simulink model "Dyn_Nonlinear_four"  (R2021a)
(part 4 of 7)

C(5,3) = 0.056*thetad2*cos(theta5)^2 - 0.028*thetad3 - 0.028*thetad4 - 0.028*thetad2 + 0.056*thetad3*cos(theta5)^2 + 0.056*thetad4*cos(theta5)^2 - 0.0098*thetad5*cos(theta5) + 0.049*thetad5*sin(theta5) + 0.14*thetad2*cos(theta4)*cos(theta5) + 0.14*thetad3*cos(theta4)*cos(theta5) + 0.07*thetad4*cos(theta4)*cos(theta5) + 0.028*thetad2*cos(theta4)*sin(theta5) - 0.1344*thetad2*cos(theta5)*sin(theta5) + 0.028*thetad3*cos(theta4)*sin(theta5) - 0.1344*thetad3*cos(theta5)*sin(theta5) + 0.014*thetad4*cos(theta4)*sin(theta5) - 0.1344*thetad4*cos(theta5)*sin(theta5) + 0.014*thetad5*cos(theta5)*sin(theta4) - 0.07*thetad5*sin(theta4)*sin(theta5) + 0.07*thetad2*cos(theta3)*cos(theta4)*cos(theta5) - 0.0672*thetad1*cos(theta2)*cos(theta3)*sin(theta4) - 0.0672*thetad1*cos(theta2)*cos(theta4)*sin(theta3) - 0.0672*thetad1*cos(theta3)*cos(theta4)*sin(theta2) - 0.014*thetad1*cos(theta2)*cos(theta5)*sin(theta3) - 0.014*thetad1*cos(theta3)*cos(theta5)*sin(theta2) + 0.014*thetad2*cos(theta3)*cos(theta4)*sin(theta5) + 0.07*thetad1*cos(theta2)*sin(theta3)*sin(theta5) + 0.07*thetad1*cos(theta3)*sin(theta2)*sin(theta5) - 0.07*thetad2*cos(theta5)*sin(theta3)*sin(theta4) + 0.0672*thetad1*sin(theta2)*sin(theta3)*sin(theta4) - 0.014*thetad2*sin(theta3)*sin(theta4)*sin(theta5) - 0.0098*thetad1*cos(theta2)*cos(theta3)*cos(theta4)*cos(theta5) + 0.049*thetad1*cos(theta2)*cos(theta3)*cos(theta4)*sin(theta5) + 0.0098*thetad1*cos(theta2)*cos(theta5)*sin(theta3)*sin(theta4) + 0.0098*thetad1*cos(theta3)*cos(theta5)*sin(theta2)*sin(theta4) + 0.0098*thetad1*cos(theta4)*cos(theta5)*sin(theta2)*sin(theta3) - 0.049*thetad1*cos(theta2)*sin(theta3)*sin(theta4)*sin(theta5) - 0.049*thetad1*cos(theta3)*sin(theta2)*sin(theta4)*sin(theta5) - 0.049*thetad1*cos(theta4)*sin(theta2)*sin(theta3)*sin(theta5) + 0.1344*thetad1*cos(theta2)*cos(theta3)*cos(theta5)^2*sin(theta4) + 0.1344*thetad1*cos(theta2)*cos(theta4)*cos(theta5)^2*sin(theta3) + 0.1344*thetad1*cos(theta3)*cos(theta4)*cos(theta5)^2*sin(theta2) - 0.1344*thetad1*cos(theta5)^2*sin(theta2)*sin(theta3)*sin(theta4) + 0.056*thetad1*cos(theta2)*cos(theta3)*cos(theta5)*sin(theta4)*sin(theta5) + 0.056*thetad1*cos(theta2)*cos(theta4)*cos(theta5)*sin(theta3)*sin(theta5) + 0.056*thetad1*cos(theta3)*cos(theta4)*cos(theta5)*sin(theta2)*sin(theta5) - 0.056*thetad1*cos(theta5)*sin(theta2)*sin(theta3)*sin(theta4)*sin(theta5) ;
C(5,4) = 0.056*thetad2*cos(theta5)^2 - 0.028*thetad3 - 0.028*thetad4 - 0.028*thetad2 + 0.056*thetad3*cos(theta5)^2 + 0.056*thetad4*cos(theta5)^2 - 0.0098*thetad5*cos(theta5) + 0.049*thetad5*sin(theta5) + 0.07*thetad2*cos(theta4)*cos(theta5) + 0.07*thetad3*cos(theta4)*cos(theta5) + 0.014*thetad2*cos(theta4)*sin(theta5) - 0.1344*thetad2*cos(theta5)*sin(theta5) + 0.014*thetad3*cos(theta4)*sin(theta5) - 0.1344*thetad3*cos(theta5)*sin(theta5) - 0.1344*thetad4*cos(theta5)*sin(theta5) + 0.07*thetad2*cos(theta3)*cos(theta4)*cos(theta5) - 0.0672*thetad1*cos(theta2)*cos(theta3)*sin(theta4) - 0.0672*thetad1*cos(theta2)*cos(theta4)*sin(theta3) - 0.0672*thetad1*cos(theta3)*cos(theta4)*sin(theta2) + 0.014*thetad2*cos(theta3)*cos(theta4)*sin(theta5) - 0.07*thetad2*cos(theta5)*sin(theta3)*sin(theta4) + 0.0672*thetad1*sin(theta2)*sin(theta3)*sin(theta4) - 0.014*thetad2*sin(theta3)*sin(theta4)*sin(theta5) - 0.0098*thetad1*cos(theta2)*cos(theta3)*cos(theta4)*cos(theta5) + 0.049*thetad1*cos(theta2)*cos(theta3)*cos(theta4)*sin(theta5) + 0.0098*thetad1*cos(theta2)*cos(theta5)*sin(theta3)*sin(theta4) + 0.0098*thetad1*cos(theta3)*cos(theta5)*sin(theta2)*sin(theta4) + 0.0098*thetad1*cos(theta4)*cos(theta5)*sin(theta2)*sin(theta3) - 0.049*thetad1*cos(theta2)*sin(theta3)*sin(theta4)*sin(theta5) - 0.049*thetad1*cos(theta3)*sin(theta2)*sin(theta4)*sin(theta5) - 0.049*thetad1*cos(theta4)*sin(theta2)*sin(theta3)*sin(theta5) + 0.1344*thetad1*cos(theta2)*cos(theta3)*cos(theta5)^2*sin(theta4) + 0.1344*thetad1*cos(theta2)*cos(theta4)*cos(theta5)^2*sin(theta3) + 0.1344*thetad1*cos(theta3)*cos(theta4)*cos(theta5)^2*sin(theta2) - 0.1344*thetad1*cos(theta5)^2*sin(theta2)*sin(theta3)*sin(theta4) + 0.056*thetad1*cos(theta2)*cos(theta3)*cos(theta5)*sin(theta4)*sin(theta5) + 0.056*thetad1*cos(theta2)*cos(theta4)*cos(theta5)*sin(theta3)*sin(theta5) + 0.056*thetad1*cos(theta3)*cos(theta4)*cos(theta5)*sin(theta2)*sin(theta5) - 0.056*thetad1*cos(theta5)*sin(theta2)*sin(theta3)*sin(theta4)*sin(theta5) ;
C(5,5) = 0.049*thetad2*sin(theta5) - 0.0098*thetad3*cos(theta5) - 0.0098*thetad4*cos(theta5) - 0.0098*thetad2*cos(theta5) + 0.049*thetad3*sin(theta5) + 0.049*thetad4*sin(theta5) + 0.07*thetad1*cos(theta2)*cos(theta5) + 0.014*thetad1*cos(theta2)*sin(theta5) + 0.014*thetad2*cos(theta5)*sin(theta4) + 0.014*thetad3*cos(theta5)*sin(theta4) - 0.07*thetad2*sin(theta4)*sin(theta5) - 0.07*thetad3*sin(theta4)*sin(theta5) + 0.07*thetad1*cos(theta2)*cos(theta3)*cos(theta5) + 0.014*thetad1*cos(theta2)*cos(theta3)*sin(theta5) + 0.014*thetad2*cos(theta3)*cos(theta5)*sin(theta4) + 0.014*thetad2*cos(theta4)*cos(theta5)*sin(theta3) - 0.07*thetad1*cos(theta5)*sin(theta2)*sin(theta3) - 0.07*thetad2*cos(theta3)*sin(theta4)*sin(theta5) - 0.07*thetad2*cos(theta4)*sin(theta3)*sin(theta5) - 0.014*thetad1*sin(theta2)*sin(theta3)*sin(theta5) - 0.049*thetad1*cos(theta2)*cos(theta3)*cos(theta5)*sin(theta4) - 0.049*thetad1*cos(theta2)*cos(theta4)*cos(theta5)*sin(theta3) - 0.049*thetad1*cos(theta3)*cos(theta4)*cos(theta5)*sin(theta2) - 0.0098*thetad1*cos(theta2)*cos(theta3)*sin(theta4)*sin(theta5) - 0.0098*thetad1*cos(theta2)*cos(theta4)*sin(theta3)*sin(theta5) - 0.0098*thetad1*cos(theta3)*cos(theta4)*sin(theta2)*sin(theta5) + 0.049*thetad1*cos(theta5)*sin(theta2)*sin(theta3)*sin(theta4) + 0.0098*thetad1*sin(theta2)*sin(theta3)*sin(theta4)*sin(theta5) ;


G=zeros(5,1);
G(1) = 0.0 ;
G(2) = 10.922454*cos(theta2) - 2.018898*sin(theta2) + 8.5347*cos(theta2)*cos(theta3) - 3.076416*cos(theta2)*sin(theta3) - 3.076416*cos(theta3)*sin(theta2) - 8.5347*sin(theta2)*sin(theta3) - 1.634346*cos(theta2)*sin(theta3)*sin(theta4) - 1.634346*cos(theta3)*sin(theta2)*sin(theta4) - 1.634346*cos(theta4)*sin(theta2)*sin(theta3) + 3.941658*sin(theta2)*sin(theta3)*sin(theta4) + 1.634346*cos(theta2)*cos(theta3)*cos(theta4) - 3.941658*cos(theta2)*cos(theta3)*sin(theta4) - 3.941658*cos(theta2)*cos(theta4)*sin(theta3) - 3.941658*cos(theta3)*cos(theta4)*sin(theta2) + 0.27468*cos(theta2)*cos(theta3)*cos(theta4)*cos(theta5) - 1.3734*cos(theta2)*cos(theta3)*cos(theta4)*sin(theta5) - 0.27468*cos(theta2)*cos(theta5)*sin(theta3)*sin(theta4) - 0.27468*cos(theta3)*cos(theta5)*sin(theta2)*sin(theta4) - 0.27468*cos(theta4)*cos(theta5)*sin(theta2)*sin(theta3) + 1.3734*cos(theta2)*sin(theta3)*sin(theta4)*sin(theta5) + 1.3734*cos(theta3)*sin(theta2)*sin(theta4)*sin(theta5) + 1.3734*cos(theta4)*sin(theta2)*sin(theta3)*sin(theta5) ;
G(3) = 8.5347*cos(theta2)*cos(theta3) - 3.076416*cos(theta2)*sin(theta3) - 3.076416*cos(theta3)*sin(theta2) - 8.5347*sin(theta2)*sin(theta3) - 1.634346*cos(theta2)*sin(theta3)*sin(theta4) - 1.634346*cos(theta3)*sin(theta2)*sin(theta4) - 1.634346*cos(theta4)*sin(theta2)*sin(theta3) + 3.941658*sin(theta2)*sin(theta3)*sin(theta4) + 1.634346*cos(theta2)*cos(theta3)*cos(theta4) - 3.941658*cos(theta2)*cos(theta3)*sin(theta4) - 3.941658*cos(theta2)*cos(theta4)*sin(theta3) - 3.941658*cos(theta3)*cos(theta4)*sin(theta2) + 0.27468*cos(theta2)*cos(theta3)*cos(theta4)*cos(theta5) - 1.3734*cos(theta2)*cos(theta3)*cos(theta4)*sin(theta5) - 0.27468*cos(theta2)*cos(theta5)*sin(theta3)*sin(theta4) - 0.27468*cos(theta3)*cos(theta5)*sin(theta2)*sin(theta4) - 0.27468*cos(theta4)*cos(theta5)*sin(theta2)*sin(theta3) + 1.3734*cos(theta2)*sin(theta3)*sin(theta4)*sin(theta5) + 1.3734*cos(theta3)*sin(theta2)*sin(theta4)*sin(theta5) + 1.3734*cos(theta4)*sin(theta2)*sin(theta3)*sin(theta5) ;
G(4) = 3.941658*sin(theta2)*sin(theta3)*sin(theta4) - 1.634346*cos(theta3)*sin(theta2)*sin(theta4) - 1.634346*cos(theta4)*sin(theta2)*sin(theta3) - 1.634346*cos(theta2)*sin(theta3)*sin(theta4) + 1.634346*cos(theta2)*cos(theta3)*cos(theta4) - 3.941658*cos(theta2)*cos(theta3)*sin(theta4) - 3.941658*cos(theta2)*cos(theta4)*sin(theta3) - 3.941658*cos(theta3)*cos(theta4)*sin(theta2) + 0.27468*cos(theta2)*cos(theta3)*cos(theta4)*cos(theta5) - 1.3734*cos(theta2)*cos(theta3)*cos(theta4)*sin(theta5) - 0.27468*cos(theta2)*cos(theta5)*sin(theta3)*sin(theta4) - 0.27468*cos(theta3)*cos(theta5)*sin(theta2)*sin(theta4) - 0.27468*cos(theta4)*cos(theta5)*sin(theta2)*sin(theta3) + 1.3734*cos(theta2)*sin(theta3)*sin(theta4)*sin(theta5) + 1.3734*cos(theta3)*sin(theta2)*sin(theta4)*sin(theta5) + 1.3734*cos(theta4)*sin(theta2)*sin(theta3)*sin(theta5) ;
G(5) = 1.3734*cos(theta5)*sin(theta2)*sin(theta3)*sin(theta4) - 1.3734*cos(theta2)*cos(theta4)*cos(theta5)*sin(theta3) - 1.3734*cos(theta3)*cos(theta4)*cos(theta5)*sin(theta2) - 0.27468*cos(theta2)*cos(theta3)*sin(theta4)*sin(theta5) - 0.27468*cos(theta2)*cos(theta4)*sin(theta3)*sin(theta5) - 0.27468*cos(theta3)*cos(theta4)*sin(theta2)*sin(theta5) - 1.3734*cos(theta2)*cos(theta3)*cos(theta5)*sin(theta4) + 0.27468*sin(theta2)*sin(theta3)*sin(theta4)*sin(theta5) ;

tau = M*a_teta+C*td+G;

return
